simulink model "New_Control_Law_I_3Axis"  (R2016a)
settings: configuration reference "AR_Drone_ConfigSet" (kept outside this file)
values from neighbouring files (symbols this model uses):
  Accel_Calib_Gain = Simulink.Parameter    [AR_DRONE_SCRIPT.m]
  Accel_Calib_Offset = Simulink.Parameter    [AR_DRONE_SCRIPT.m]
undefined symbols (not defined in the file or in its folder): Drone_StateModeType, Mag_Calib_Gain_Vector, Mag_Calib_Offset_Vector, Navigation, Navigation_KF_Lib, sigbuilder_block
libraries: simulink x16, vrlib x7, aerolibtransform2 x5, AR_Drone_Sensors x2, AR_Drone_Actuators x2, aerolibutil x2, dspnetwork x2
(part 2 of 3)

== system New_Control_Law_I_3Axis/Flight Controller/Supervisory Flight Controller/Attitude_Control/Yaw Counter-Active Control ==
  note: This Yaw Controller will prevent the drone from
      | rotating but does not tell the drone to rotate to a specified angle
  Euler_Yaw_Deg : Inport
  Rate_Gyro_R_deg : Inport  Port=2
  "Desired_yaw " : Inport  Port=3
  Add1 : Sum  Inputs=+-  AccumDataTypeStr=single  OutDataTypeStr=single
  Add2 : Sum  Inputs=+-  AccumDataTypeStr=single  OutDataTypeStr=single
  Data Type Conversion : DataTypeConversion  OutDataTypeStr=int16
  Discrete Derivative : simulink/Discrete/Discrete Derivative  gainval=1.0  ICPrevScaledInput=0.0  InputProcessing=Inherited  OutMin=[]  OutMax=[]  OutDataType=fixdt(1, 16)  OutScaling=2^-10  DoSatur=off
  InterChange_Axis : Gain  Gain=-1  ParamDataTypeStr=single  OutDataTypeStr=single
      settings: AttributesFormatString=%<Gain>
  To Degrees2 : Gain  Gain=180/pi  ParamDataTypeStr=single  OutDataTypeStr=single
      settings: AttributesFormatString=%<Gain>
  To Degrees3 : Gain  ParamDataTypeStr=single  OutDataTypeStr=single
      settings: AttributesFormatString=%<Gain>
  Yaw_contribution : Gain  Gain=2.5*2  ParamDataTypeStr=single  OutDataTypeStr=single
      settings: AttributesFormatString=%<Gain>
  Yaw_contribution1 : Gain  Gain=0.04  ParamDataTypeStr=single  OutDataTypeStr=single
      settings: AttributesFormatString=%<Gain>
  YawCommand : Outport
  wires:
  Yaw_contribution1/1 -> Data Type Conversion/1
  To Degrees3/1 -> Add1/2
  Euler_Yaw_Deg/1 -> InterChange_Axis/1
  Add1/1 -> Yaw_contribution1/1
  Yaw_contribution/1 -> Add1/1
  Add2/1 -> Yaw_contribution/1
  InterChange_Axis/1 -> Discrete Derivative/1
  Discrete Derivative/1 -> Add2/1
  To Degrees2/1 -> Add2/2
  "Desired_yaw "/1 -> To Degrees2/1
  Rate_Gyro_R_deg/1 -> To Degrees3/1
  Data Type Conversion/1 -> YawCommand/1

== system New_Control_Law_I_3Axis/Flight Controller/Supervisory Flight Controller/Attitude_Control/Yaw Signal Builder  ==
  Demux : Demux  Tag=STV Demux  Outputs=1
  FromWs : FromWorkspace  Tag=STV FromWs  VariableName=tuvar
      SigBuilderData=|
      | common.afterFinalStr = 'Extrapolate'
      | common.sampleTime = '-1'
      | dataSet.timeRange = [0 20]
      | dataSet.name = 'Group 1'
      | sbobj.Groups.Name = 'Group 1'
      | sbobj.Groups.Signals.Name = 'Signal 1'
      | sbobj.Groups.Signals.XData = [0 10 10 12.5 12.5 15 15 20]
      | sbobj.Groups.Signals.YData = [0 0 2 2 -2 -2 0 0]
      | sbobj.Groups.TimeRange = [0 20]
  Signal 1 : Outport  Tag=STV Outport
  wires:
  Demux/1 -> Signal 1/1
  FromWs/1 -> Demux/1

== system New_Control_Law_I_3Axis/Navigation/CheckSum Pre-Processing/Accelerometer Processing ==
  Raw Data : Inport
  CheckSum Flag : Inport  Port=2
  Holding Value : Inport  Port=3
  Calculate Accel Data : Subsystem  Commented=through
  CheckSum Correction : Subsystem
  Processed Data : Outport
  wires:
  Holding Value/1 -> CheckSum Correction/3(Holding Value)
  Calculate Accel Data/1(Processed Accel Data) -> CheckSum Correction/1(CalculatedData)
  CheckSum Correction/1(Pre-Processed Height) -> Processed Data/1
  Raw Data/1 -> Calculate Accel Data/1(Raw Accel Data)
  CheckSum Flag/1 -> CheckSum Correction/2(CheckSumFlag)

== system New_Control_Law_I_3Axis/Navigation/CheckSum Pre-Processing/Magnetometer ==
  Magnetometer : Inport
  CheckSum Flag : Inport  Port=2
  Holding Value : Inport  Port=3
  CheckSum Correction : Subsystem
  Process Raw Mag Data : Subsystem  Commented=through
  Processed Data : Outport
  wires:
  Holding Value/1 -> CheckSum Correction/3(Holding Value)
  Process Raw Mag Data/1(ProcessedData) -> CheckSum Correction/1(CalculatedData)
  Magnetometer/1 -> Process Raw Mag Data/1(Magnetometer)
  CheckSum Correction/1(Pre-Processed Data) -> Processed Data/1
  CheckSum Flag/1 -> CheckSum Correction/2(CheckSumFlag)

== system New_Control_Law_I_3Axis/Navigation/CheckSum Pre-Processing/RateGyro Processing ==
  Raw Data : Inport
  CheckSum Flag : Inport  Port=2
  Holding Value : Inport  Port=3
  CheckSum Correction : Subsystem
  Process Data : Subsystem  Commented=through
  Processed Data : Outport
  wires:
  Holding Value/1 -> CheckSum Correction/3(Holding Value)
  Process Data/1(Processed Data) -> CheckSum Correction/1(CalculatedData)
  Raw Data/1 -> Process Data/1(Raw Data)
  CheckSum Correction/1(Pre-Processed Height) -> Processed Data/1
  CheckSum Flag/1 -> CheckSum Correction/2(CheckSumFlag)

== system New_Control_Law_I_3Axis/Navigation/CheckSum Pre-Processing/TempFilter ==
  Magnetometer : Inport
  CheckSum Flag : Inport  Port=2
  HoldingValue : Inport  Port=3
  CheckSum Correction : Subsystem
  Process Raw Mag Data : Subsystem  Commented=through
  Processed Data : Outport
  wires:
  HoldingValue/1 -> CheckSum Correction/3(Holding Value)
  Process Raw Mag Data/1(ProcessedData) -> CheckSum Correction/1(CalculatedData)
  Magnetometer/1 -> Process Raw Mag Data/1(Magnetometer)
  CheckSum Correction/1(Pre-Processed Data) -> Processed Data/1
  CheckSum Flag/1 -> CheckSum Correction/2(CheckSumFlag)

== system New_Control_Law_I_3Axis/Navigation/CheckSum Pre-Processing/Ultrasound Processing ==
  note: '192.168.1.1' 1 17725
  Raw Ultrasound : Inport
  CheckSum Flag : Inport  Port=2
  Holding Value : Inport  Port=3
  CheckSum Correction : Subsystem
  Data Type Conversion1 : DataTypeConversion
  Delay1 : Delay  DelayLength=1  InitialCondition=0
  Height Calculation : MATLAB Function  TreatAsAtomicUnit=on
  Saturation1 : Saturate  UpperLimit=100e3  LowerLimit=0
  Processed Data : Outport
  wires:
  Holding Value/1 -> CheckSum Correction/3(Holding Value)
  Saturation1/1 -> Processed Data/1
  CheckSum Correction/1(Pre-Processed Height) -> Saturation1/1
  CheckSum Flag/1 -> CheckSum Correction/2(CheckSumFlag)
  Height Calculation/1(y) -> CheckSum Correction/1(CalculatedData)
  Raw Ultrasound/1 -> Data Type Conversion1/1
  Height Calculation/2(prev_good_height) -> Delay1/1
  Data Type Conversion1/1 -> Height Calculation/1(u)
  Delay1/1 -> Height Calculation/2(z_1)

== system New_Control_Law_I_3Axis/Navigation/Data Conversion and Measurement Calculation/Calculate Gravity Vector ==
  Accel : Inport
  Accel_Offset : Inport  Port=2
  Accelerometer Neutral Gain and Offset : Subsystem
  Calibration_GainOffset : Subsystem
  Compare Calibration : Scope  NumInputPorts=2
  Compare Filter : Scope  NumInputPorts=2
  Compare Offset : Scope  NumInputPorts=2
  InitialCondition_Offset : Subsystem
  Low Pass Filter : Subsystem
  Normalize Vector : vrlib/Utilities/Normalize Vector  maxzero=0
  Accel_Norm : Outport
  wires:
  Accel_Offset/1 -> InitialCondition_Offset/2(Accel_Offset)
  Accelerometer Neutral Gain and Offset/1(Processed Accel Data) -> Compare Calibration/2, Calibration_GainOffset/1(Pre)
  Calibration_GainOffset/1(Post) -> Compare Offset/2, Compare Calibration/1, InitialCondition_Offset/1(Pre)
  Low Pass Filter/1(Filtered Accel) -> Normalize Vector/1, Compare Filter/1
  InitialCondition_Offset/1(Post) -> Low Pass Filter/1(Offset Accel), Compare Filter/2, Compare Offset/1
  Accel/1 -> Accelerometer Neutral Gain and Offset/1(Raw Accel Data)
  Normalize Vector/1 -> Accel_Norm/1

== system New_Control_Law_I_3Axis/Navigation/Data Conversion and Measurement Calculation/Calibration_Scale_and_Offset ==
  RawMag : Inport
  Normalize Vector : vrlib/Utilities/Normalize Vector  maxzero=0
  Process Raw Mag Data : Subsystem  Variant=on  OverrideUsingVariant=TempVariantA
  Normalized  Magnetometer : Outport
  wires:
  Process Raw Mag Data/1(MagVector) -> Normalize Vector/1
  RawMag/1 -> Process Raw Mag Data/1(Magnetometer)
  Normalize Vector/1 -> Normalized  Magnetometer/1

== system New_Control_Law_I_3Axis/Navigation/Data Conversion and Measurement Calculation/Remove Offset ==
  Raw Gyro Values : Inport
  Gyro Offset : Inport  Port=2
  BeforeAfter : Scope
  Demux : Demux  Outputs=3
  Demux1 : Demux  Outputs=3
  Display : Display
  Mux : Mux  Inputs=2
  Mux1 : Mux  Inputs=3
  Process Raw Rate Gyro Data : Subsystem
  Sum : Sum  Inputs=|+-
  Sum1 : Sum  Inputs=|+-
  Sum2 : Sum  Inputs=|+-
  Gyro Offset Remove : Outport
  tag scope: GyroOffset_Tag=global
  wires:
  Process Raw Rate Gyro Data/1(Processed Data) -> Gyro Offset Remove/1
  Mux/1 -> BeforeAfter/1
  Raw Gyro Values/1 -> Demux/1, Mux/1, [GyroOffset_Tag]
  Gyro Offset/1 -> Demux1/1
  Mux1/1 -> Process Raw Rate Gyro Data/1(Raw Rate Gyro Data), Display/1, Mux/2
  Demux1/3 -> Sum2/2
  Demux1/2 -> Sum1/2
  Demux1/1 -> Sum/2
  Demux/2 -> Sum1/1
  Demux/1 -> Sum/1
  Sum1/1 -> Mux1/2
  Demux/3 -> Sum2/1
  Sum2/1 -> Mux1/3
  Sum/1 -> Mux1/1

== system New_Control_Law_I_3Axis/Navigation/SL3D Visualization/Interchange Axes Accel for SL3D  ==
  VRML_in : Inport
  Demux1 : Demux  Outputs=3
  Gain1 : Gain  Gain=3
  Gain2 : Gain
  Gain3 : Gain
  Mux2 : Mux  Inputs=3
  VRML_out : Outport
  wires:
  VRML_in/1 -> Gain1/1
  Demux1/2 -> Gain2/1
  Mux2/1 -> VRML_out/1
  Gain3/1 -> Mux2/3
  Gain2/1 -> Mux2/1
  Demux1/3 -> Mux2/2
  Demux1/1 -> Gain3/1
  Gain1/1 -> Demux1/1

== system New_Control_Law_I_3Axis/Navigation/SL3D Visualization/Interchange Axes Mag for SL3D  ==
  VRML_in : Inport
  Home Drone : Subsystem
  Subsystem : Subsystem  Commented=on
  Work Drone : Subsystem
  Work Drone - supposed work drone .. not really : Subsystem
  VRML_out : Outport
  wires:
  Work Drone/1(Out1) -> VRML_out/1
  VRML_in/1 -> Home Drone/1(In1), Work Drone/1(In1)

== system New_Control_Law_I_3Axis/Navigation/SL3D Visualization/Interchange Axis Mag Project for SL3D ==
  VRML_in : Inport
  Demux1 : Demux  Outputs=3
  Gain2 : Gain
  Gain3 : Gain
  Mux2 : Mux  Inputs=3
  VRML_out : Outport
  wires:
  Demux1/2 -> Gain2/1
  Mux2/1 -> VRML_out/1
  Gain3/1 -> Mux2/3
  Gain2/1 -> Mux2/1
  Demux1/3 -> Mux2/2
  Demux1/1 -> Gain3/1
  VRML_in/1 -> Demux1/1

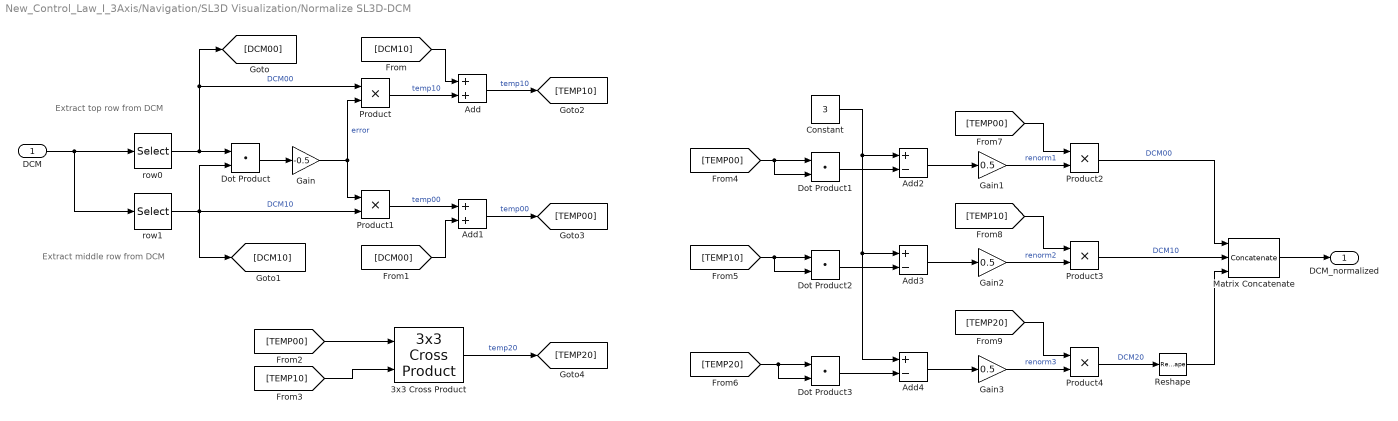
== system New_Control_Law_I_3Axis/Navigation/SL3D Visualization/Normalize SL3D-DCM ==
  note: Extract top row from DCM
  note: Extract middle row from DCM
  DCM : Inport  OutDataTypeStr=double  PortDimensions=[3,3]
  3x3 Cross Product : aerolibutil/3x3 Cross Product
  Add : Sum
  Add1 : Sum
  Add2 : Sum  Inputs=+-
  Add3 : Sum  Inputs=+-
  Add4 : Sum  Inputs=+-
  Constant : Constant  Value=3  OutDataTypeStr=double  SampleTime=-1
  Dot Product{,1..3} (4 alike) : DotProduct  InputSameDT=on  OutDataTypeStr=Inherit: Inherit via internal rule
  Gain : Gain  Gain=-0.5
  Gain1 : Gain  Gain=0.5  OutDataTypeStr=single
  Gain2 : Gain  Gain=0.5  OutDataTypeStr=single
  Gain3 : Gain  Gain=0.5  OutDataTypeStr=single
  Matrix Concatenate : Concatenate  NumInputs=3  Mode=Multidimensional array
  Product{,1..4} (5 alike) : Product  RndMeth=Zero
  Reshape : Reshape  OutputDimensionality=Row vector (2-D)
  row0 : Selector  NumberOfDimensions=2  IndexMode=Zero-based  InputPortWidth=3  IndexOptions=Index vector (dialog),Index vector (dialog)  Indices=0,[0:2]  OutputSizes=1,1
  row1 : Selector  NumberOfDimensions=2  IndexMode=Zero-based  InputPortWidth=3  IndexOptions=Index vector (dialog),Index vector (dialog)  Indices=1,[0:2]  OutputSizes=1,1
  DCM_normalized : Outport  OutDataTypeStr=double
  wires:
  DCM/1 -> row0/1, row1/1
  row0/1 -> Dot Product/1, Product/1, [DCM00]  "DCM00"
  row1/1 -> Dot Product/2, Product1/2, [DCM10]  "DCM10"
  Dot Product/1 -> Gain/1
  Gain/1 -> Product/2, Product1/1  "error"
  Product/1 -> Add/2  "temp10"
  Product1/1 -> Add1/1  "temp00"
  [DCM10] -> Add/1
  [DCM00] -> Add1/2
  Add/1 -> [TEMP10]  "temp10"
  Add1/1 -> [TEMP00]  "temp00"
  3x3 Cross Product/1 -> [TEMP20]  "temp20"
  [TEMP00] -> 3x3 Cross Product/1
  [TEMP10] -> 3x3 Cross Product/2
  [TEMP00] -> Dot Product1/1, Dot Product1/2
  [TEMP10] -> Dot Product2/1, Dot Product2/2
  [TEMP20] -> Dot Product3/1, Dot Product3/2
  Dot Product1/1 -> Add2/2
  Constant/1 -> Add2/1, Add4/1, Add3/1
  Add2/1 -> Gain1/1
  Gain1/1 -> Product2/2  "renorm1"
  Add3/1 -> Gain2/1
  Gain2/1 -> Product3/2  "renorm2"
  Dot Product2/1 -> Add3/2
  Add4/1 -> Gain3/1
  Gain3/1 -> Product4/2  "renorm3"
  Dot Product3/1 -> Add4/2
  [TEMP00] -> Product2/1
  [TEMP10] -> Product3/1
  [TEMP20] -> Product4/1
  Product2/1 -> Matrix Concatenate/1  "DCM00"
  Product3/1 -> Matrix Concatenate/2  "DCM10"
  Product4/1 -> Reshape/1  "DCM20"
  Matrix Concatenate/1 -> DCM_normalized/1
  Reshape/1 -> Matrix Concatenate/3

== system New_Control_Law_I_3Axis/Navigation/SL3D Visualization/SL3D DCM Output - used to adjust axes to fit wit SL3D convention ==

== system New_Control_Law_I_3Axis/SL3D Visualization/Interchange Axes Mag for SL3D /Home Drone ==
  note: z
  note: x
  note: y
  note: This comes close, however, it doesnt seem that the axis changes properly
      | ie: i rotate drone, the green dot follows it. This  tells me the Z-axis is not
      |  properly placed
  In1 : Inport
  Demux1 : Demux  Outputs=3
  Gain : Gain  Gain=-1
  Gain1 : Gain
  Gain2 : Gain
  Mux2 : Mux  Inputs=3
  Out1 : Outport
  wires:
  Gain1/1 -> Mux2/1
  Demux1/2 -> Gain1/1
  Gain/1 -> Mux2/3
  Demux1/1 -> Gain/1
  Gain2/1 -> Mux2/2
  Demux1/3 -> Gain2/1
  In1/1 -> Demux1/1
  Mux2/1 -> Out1/1

== system New_Control_Law_I_3Axis/SL3D Visualization/Interchange Axes Mag for SL3D /Subsystem ==
  note: z
  note: x
  note: y
  note: This comes close, however, it doesnt seem that the axis changes properly
      | ie: i rotate drone, the green dot follows it. This  tells me the Z-axis is not
      |  properly placed
  In1 : Inport
  Demux1 : Demux  Outputs=3
  Gain : Gain
  Gain1 : Gain  Gain=-1
  Gain2 : Gain  Gain=-1
  Mux2 : Mux  Inputs=3
  Out1 : Outport
  wires:
  In1/1 -> Demux1/1
  Demux1/3 -> Gain/1
  Demux1/2 -> Gain1/1
  Mux2/1 -> Out1/1
  Gain1/1 -> Mux2/1
  Gain/1 -> Mux2/3
  Gain2/1 -> Mux2/2
  Demux1/1 -> Gain2/1

== system New_Control_Law_I_3Axis/SL3D Visualization/Interchange Axes Mag for SL3D /Work Drone ==
  note: z
  note: x
  note: y
  note: This comes close, however, it doesnt seem that the axis changes properly
      | ie: i rotate drone, the green dot follows it. This  tells me the Z-axis is not
      |  properly placed
  In1 : Inport
  Demux1 : Demux  Outputs=3
  Gain : Gain  Gain=-1
  Gain1 : Gain
  Gain2 : Gain
  Mux2 : Mux  Inputs=3
  Out1 : Outport
  wires:
  Gain1/1 -> Mux2/1
  Demux1/2 -> Gain1/1
  Gain/1 -> Mux2/3
  Demux1/1 -> Gain/1
  Gain2/1 -> Mux2/2
  Demux1/3 -> Gain2/1
  In1/1 -> Demux1/1
  Mux2/1 -> Out1/1

== system New_Control_Law_I_3Axis/SL3D Visualization/Interchange Axes Mag for SL3D /Work Drone - supposed work drone .. not really ==
  note: z
  note: x
  note: y
  note: This comes close, however, it doesnt seem that the axis changes properly
      | ie: i rotate drone, the green dot follows it. This  tells me the Z-axis is not
      |  properly placed
  In1 : Inport
  Demux1 : Demux  Outputs=3
  Gain : Gain  Gain=-1
  Gain1 : Gain
  Gain2 : Gain  Gain=-1
  Mux2 : Mux  Inputs=3
  Out1 : Outport
  wires:
  Gain1/1 -> Mux2/1
  Demux1/2 -> Gain1/1
  Gain/1 -> Mux2/3
  Demux1/1 -> Gain/1
  Gain2/1 -> Mux2/2
  Demux1/3 -> Gain2/1
  In1/1 -> Demux1/1
  Mux2/1 -> Out1/1

== system New_Control_Law_I_3Axis/Sensor  Telemetry/CheckSum_Correct_Pressure/CheckSum Correction ==
  CalculatedData : Inport
  CheckSumFlag : Inport  Port=2
  Holding Value : Inport  Port=3
  Compare To Zero : simulink/Logic and Bit Operations/Compare To Zero  relop=>  OutDataTypeStr=boolean
  Delay : Delay  DelayLength=3  InitialCondition=0
  Generate Sample Holding Pulse : Subsystem
  "If True, we have good data, If false, we have bad data, With bad data, use previous good data from N samples ago and hold it on that value for M samples" : Switch  Criteria=u2 > Threshold
  Invert Logic : Logic  Operator=NOT  AllPortsSameDT=off  OutDataTypeStr=boolean
  Logical Operator1 : Logic  Operator=NOT  AllPortsSameDT=off  OutDataTypeStr=boolean
  Pre-Processed Height : Outport
  wires:
  CheckSumFlag/1 -> Compare To Zero/1
  CalculatedData/1 -> "If True, we have good data, If false, we have bad data, With bad data, use previous good data from N samples ago and hold it on that value for M samples"/1
  "If True, we have good data, If false, we have bad data, With bad data, use previous good data from N samples ago and hold it on that value for M samples"/1 -> Pre-Processed Height/1, Delay/1
  Delay/1 -> "If True, we have good data, If false, we have bad data, With bad data, use previous good data from N samples ago and hold it on that value for M samples"/3
  Compare To Zero/1 -> Logical Operator1/1
  Generate Sample Holding Pulse/1(Hold_Data_Pulse) -> Invert Logic/1
  Logical Operator1/1 -> Generate Sample Holding Pulse/1(CheckSumFlag)
  Invert Logic/1 -> "If True, we have good data, If false, we have bad data, With bad data, use previous good data from N samples ago and hold it on that value for M samples"/2
  Holding Value/1 -> Generate Sample Holding Pulse/2(HoldDataTicks_Value)

== system New_Control_Law_I_3Axis/Sensor  Telemetry/CheckSum_Correct_Temp/CheckSum Correction ==
  CalculatedData : Inport
  CheckSumFlag : Inport  Port=2
  Holding Value : Inport  Port=3
  Compare To Zero : simulink/Logic and Bit Operations/Compare To Zero  relop=>  OutDataTypeStr=boolean
  Delay : Delay  DelayLength=3  InitialCondition=0
  Generate Sample Holding Pulse : Subsystem
  "If True, we have good data, If false, we have bad data, With bad data, use previous good data from N samples ago and hold it on that value for M samples" : Switch  Criteria=u2 > Threshold
  Invert Logic : Logic  Operator=NOT  AllPortsSameDT=off  OutDataTypeStr=boolean
  Logical Operator1 : Logic  Operator=NOT  AllPortsSameDT=off  OutDataTypeStr=boolean
  Pre-Processed Height : Outport
  wires:
  CheckSumFlag/1 -> Compare To Zero/1
  CalculatedData/1 -> "If True, we have good data, If false, we have bad data, With bad data, use previous good data from N samples ago and hold it on that value for M samples"/1
  "If True, we have good data, If false, we have bad data, With bad data, use previous good data from N samples ago and hold it on that value for M samples"/1 -> Pre-Processed Height/1, Delay/1
  Delay/1 -> "If True, we have good data, If false, we have bad data, With bad data, use previous good data from N samples ago and hold it on that value for M samples"/3
  Compare To Zero/1 -> Logical Operator1/1
  Generate Sample Holding Pulse/1(Hold_Data_Pulse) -> Invert Logic/1
  Logical Operator1/1 -> Generate Sample Holding Pulse/1(CheckSumFlag)
  Invert Logic/1 -> "If True, we have good data, If false, we have bad data, With bad data, use previous good data from N samples ago and hold it on that value for M samples"/2
  Holding Value/1 -> Generate Sample Holding Pulse/2(HoldDataTicks_Value)

== system New_Control_Law_I_3Axis/Sensor  Telemetry/Data Collection/Low Pass Filter ==
  GyroMeasure : Inport
  Demux : Demux  Outputs=2
  Digital Low Pass Filter1 : DiscreteTransferFcn  Numerator=[0.04877]  Denominator=[1 -0.9512]  OutDataTypeStr=int16
  Digital Low Pass Filter2 : DiscreteTransferFcn  Numerator=[0.04877]  Denominator=[1 -0.9512]  OutDataTypeStr=int16
  Digital Low Pass Filter3 : DiscreteTransferFcn  Commented=on  Numerator=[0.04877]  Denominator=[1 -0.9512]  OutDataTypeStr=int16
  Mux3 : Mux  Inputs=2
  GyroFiltered : Outport
  wires:
  Mux3/1 -> GyroFiltered/1
  Demux/1 -> Digital Low Pass Filter2/1
  GyroMeasure/1 -> Demux/1
  Demux/2 -> Digital Low Pass Filter1/1
  Digital Low Pass Filter2/1 -> Mux3/1
  Digital Low Pass Filter1/1 -> Mux3/2

== system New_Control_Law_I_3Axis/Flight Controller/Supervisory Flight Controller/Attitude_Control/Roll Pitch Controller/Low Pass Filter ==
  GyroMeasure : Inport
  Demux : Demux  Outputs=2
  Digital Low Pass Filter1 : DiscreteTransferFcn  Numerator=[0.04877]  Denominator=[1 -0.9512]  OutDataTypeStr=int16
  Digital Low Pass Filter2 : DiscreteTransferFcn  Numerator=[0.04877]  Denominator=[1 -0.9512]  OutDataTypeStr=int16
  Digital Low Pass Filter3 : DiscreteTransferFcn  Commented=on  Numerator=[0.04877]  Denominator=[1 -0.9512]  OutDataTypeStr=int16
  Mux3 : Mux  Inputs=2
  GyroFiltered : Outport
  wires:
  Mux3/1 -> GyroFiltered/1
  Demux/1 -> Digital Low Pass Filter2/1
  GyroMeasure/1 -> Demux/1
  Demux/2 -> Digital Low Pass Filter1/1
  Digital Low Pass Filter2/1 -> Mux3/1
  Digital Low Pass Filter1/1 -> Mux3/2

== system New_Control_Law_I_3Axis/Flight Controller/Supervisory Flight Controller/Attitude_Control/Roll Pitch Controller/Outer Loop Euler Angle Control Loop ==
  Attitude_Rate : Inport
  Motor Armed : Inport  Port=2
  Logical Operator : Logic  Operator=NOT  AllPortsSameDT=off  OutDataTypeStr=boolean
  PID Controller : simulink/Continuous/PID Controller  Controller=PID  TimeDomain=Discrete-time  SampleTime=-1  IntegratorMethod=Forward Euler  FilterMethod=Forward Euler  Form=Parallel  UseFilter=on  ControllerParametersSource=internal  P=2.8281  I=28.23  D=0.023379  N=0.0076593  InitialConditionSource=internal  InitialConditionForIntegrator=0  InitialConditionForFilter=0  ExternalReset=level  LimitOutput=on  UpperSaturationLimit=30  LowerSaturationLimit=-30  LinearizeAsGain=on  AntiWindupMode=clamping  Kb=1  TrackingMode=off  Kt=1  PParamMin=[]  PParamMax=[]  IParamMin=[]  IParamMax=[]  DParamMin=[]  DParamMax=[]  NParamMin=[]  NParamMax=[]  KbParamMin=[]  KbParamMax=[]  KtParamMin=[]  KtParamMax=[]  POutMin=[]  POutMax=[]  IOutMin=[]  IOutMax=[]  DOutMin=[]  DOutMax=[]  NOutMin=[]  NOutMax=[]  KbOutMin=[]  KbOutMax=[]  KtOutMin=[]  KtOutMax=[]  IntegratorOutMin=[]  IntegratorOutMax=[]  FilterOutMin=[]  FilterOutMax=[]  SumOutMin=[]  SumOutMax=[]  SumI1OutMin=[]  SumI1OutMax=[]  SumI2OutMin=[]  SumI2OutMax=[]  SumI3OutMin=[]  SumI3OutMax=[]  SumDOutMin=[]  SumDOutMax=[]  SaturationOutMin=[]  SaturationOutMax=[]  IntegratorContinuousStateAttributes=''  IntegratorStateMustResolveToSignalObject=off  IntegratorRTWStateStorageClass=Auto  FilterContinuousStateAttributes=''  FilterStateMustResolveToSignalObject=off  FilterRTWStateStorageClass=Auto  DifferentiatorICPrevScaledInput=0  DifferentiatorOutMin=[]  DifferentiatorOutMax=[]
  PID Controller1 : simulink/Continuous/PID Controller  Controller=PID  TimeDomain=Discrete-time  SampleTime=-1  IntegratorMethod=Forward Euler  FilterMethod=Forward Euler  Form=Parallel  UseFilter=on  ControllerParametersSource=internal  P=0.10084*2  I=0.13631*2  D=-0.011755  N=5  InitialConditionSource=internal  InitialConditionForIntegrator=0  InitialConditionForFilter=0  ExternalReset=level  LimitOutput=on  UpperSaturationLimit=30  LowerSaturationLimit=-30  LinearizeAsGain=on  AntiWindupMode=clamping  Kb=1  TrackingMode=off  Kt=1  PParamMin=[]  PParamMax=[]  IParamMin=[]  IParamMax=[]  DParamMin=[]  DParamMax=[]  NParamMin=[]  NParamMax=[]  KbParamMin=[]  KbParamMax=[]  KtParamMin=[]  KtParamMax=[]  POutMin=[]  POutMax=[]  IOutMin=[]  IOutMax=[]  DOutMin=[]  DOutMax=[]  NOutMin=[]  NOutMax=[]  KbOutMin=[]  KbOutMax=[]  KtOutMin=[]  KtOutMax=[]  IntegratorOutMin=[]  IntegratorOutMax=[]  FilterOutMin=[]  FilterOutMax=[]  SumOutMin=[]  SumOutMax=[]  SumI1OutMin=[]  SumI1OutMax=[]  SumI2OutMin=[]  SumI2OutMax=[]  SumI3OutMin=[]  SumI3OutMax=[]  SumDOutMin=[]  SumDOutMax=[]  SaturationOutMin=[]  SaturationOutMax=[]  IntegratorContinuousStateAttributes=''  IntegratorStateMustResolveToSignalObject=off  IntegratorRTWStateStorageClass=Auto  FilterContinuousStateAttributes=''  FilterStateMustResolveToSignalObject=off  FilterRTWStateStorageClass=Auto  DifferentiatorICPrevScaledInput=0  DifferentiatorOutMin=[]  DifferentiatorOutMax=[]
  AttitudeRateCmd : Outport
  wires:
  PID Controller1/1 -> AttitudeRateCmd/1  "AttitudeRateCmd"
  Motor Armed/1 -> Logical Operator/1
  Logical Operator/1 -> PID Controller1/2
  Attitude_Rate/1 -> PID Controller1/1

== system New_Control_Law_I_3Axis/Navigation/CheckSum Pre-Processing/Accelerometer Processing/Calculate Accel Data ==
  Raw Accel Data : Inport
  Bias : Constant  Value=[0 4096 4096]
  Gain : Gain  Gain=[0.001953125, 0.001953125, 0.001953125]
  Neutral Bias : Constant  Value=[2048 2048 2048]
  Sum : Sum  Inputs=|-+
  Sum1 : Sum  Inputs=|+-
  Processed Accel Data : Outport
  wires:
  Bias/1 -> Sum/2
  Neutral Bias/1 -> Sum1/2
  Sum/1 -> Sum1/1
  Gain/1 -> Processed Accel Data/1
  Sum1/1 -> Gain/1
  Raw Accel Data/1 -> Sum/1

== system New_Control_Law_I_3Axis/Navigation/CheckSum Pre-Processing/Accelerometer Processing/CheckSum Correction ==
  CalculatedData : Inport
  CheckSumFlag : Inport  Port=2
  Holding Value : Inport  Port=3
  Compare To Zero : simulink/Logic and Bit Operations/Compare To Zero  relop=>  OutDataTypeStr=boolean
  Delay : Delay  DelayLength=3  InitialCondition=0
  Generate Sample Holding Pulse : Subsystem
  "If True, we have good data, If false, we have bad data, With bad data, use previous good data from N samples ago and hold it on that value for M samples" : Switch  Criteria=u2 > Threshold
  Invert Logic : Logic  Operator=NOT  AllPortsSameDT=off  OutDataTypeStr=boolean
  Logical Operator1 : Logic  Operator=NOT  AllPortsSameDT=off  OutDataTypeStr=boolean
  Pre-Processed Height : Outport
  wires:
  Holding Value/1 -> Generate Sample Holding Pulse/2(HoldDataTicks_Value)
  Invert Logic/1 -> "If True, we have good data, If false, we have bad data, With bad data, use previous good data from N samples ago and hold it on that value for M samples"/2
  Logical Operator1/1 -> Generate Sample Holding Pulse/1(CheckSumFlag)
  Generate Sample Holding Pulse/1(Hold_Data_Pulse) -> Invert Logic/1
  Compare To Zero/1 -> Logical Operator1/1
  Delay/1 -> "If True, we have good data, If false, we have bad data, With bad data, use previous good data from N samples ago and hold it on that value for M samples"/3
  "If True, we have good data, If false, we have bad data, With bad data, use previous good data from N samples ago and hold it on that value for M samples"/1 -> Delay/1, Pre-Processed Height/1
  CalculatedData/1 -> "If True, we have good data, If false, we have bad data, With bad data, use previous good data from N samples ago and hold it on that value for M samples"/1
  CheckSumFlag/1 -> Compare To Zero/1

== system New_Control_Law_I_3Axis/Navigation/CheckSum Pre-Processing/Magnetometer/CheckSum Correction ==
  CalculatedData : Inport
  CheckSumFlag : Inport  Port=2
  Holding Value : Inport  Port=3
  Compare To Zero : simulink/Logic and Bit Operations/Compare To Zero  relop=>  OutDataTypeStr=boolean
  Delay : Delay  DelayLength=3  InitialCondition=0
  Generate Sample Holding Pulse : Subsystem
  "If True, we have good data, If false, we have bad data, With bad data, use previous good data from N samples ago and hold it on that value for M samples" : Switch  Criteria=u2 > Threshold
  Invert Logic : Logic  Operator=NOT  AllPortsSameDT=off  OutDataTypeStr=boolean
  Logical Operator1 : Logic  Operator=NOT  AllPortsSameDT=off  OutDataTypeStr=boolean
  Pre-Processed Data : Outport
  wires:
  Holding Value/1 -> Generate Sample Holding Pulse/2(HoldDataTicks_Value)
  Invert Logic/1 -> "If True, we have good data, If false, we have bad data, With bad data, use previous good data from N samples ago and hold it on that value for M samples"/2
  Logical Operator1/1 -> Generate Sample Holding Pulse/1(CheckSumFlag)
  Generate Sample Holding Pulse/1(Hold_Data_Pulse) -> Invert Logic/1
  Compare To Zero/1 -> Logical Operator1/1
  Delay/1 -> "If True, we have good data, If false, we have bad data, With bad data, use previous good data from N samples ago and hold it on that value for M samples"/3
  "If True, we have good data, If false, we have bad data, With bad data, use previous good data from N samples ago and hold it on that value for M samples"/1 -> Delay/1, Pre-Processed Data/1
  CalculatedData/1 -> "If True, we have good data, If false, we have bad data, With bad data, use previous good data from N samples ago and hold it on that value for M samples"/1
  CheckSumFlag/1 -> Compare To Zero/1

== system New_Control_Law_I_3Axis/Navigation/CheckSum Pre-Processing/Magnetometer/Process Raw Mag Data ==
  note: magnetometer[ 0 ] = - ( float ) navdata.mx ;
      | magnetometer[ 1 ] = ( float ) navdata.my ;
      | magnetometer[ 2 ] = - ( float ) navdata.mz ;
      | const float Sensitivity[ 3 ] = { 0.0071492608 , 0.0070882491 , 0.0074057781 } ;
      | const float Neutral[ 3 ] = { 118.0 , - 65.0 , 110.0 } ;
  Magnetometer : Inport
  Bias : Constant  Value=[ 118.0, -65.0, 110.0 ]
  Sum : Sum  Inputs=|+-
  postGain : Gain  Gain=[0.0071492608, 0.0070882491, 0.0074057781]
  preGain : Gain  Gain=[-1 1 -1]
  ProcessedData : Outport
  wires:
  Bias/1 -> Sum/2
  preGain/1 -> Sum/1
  Sum/1 -> postGain/1
  Magnetometer/1 -> preGain/1
  postGain/1 -> ProcessedData/1

== system New_Control_Law_I_3Axis/Navigation/CheckSum Pre-Processing/RateGyro Processing/CheckSum Correction ==
  CalculatedData : Inport
  CheckSumFlag : Inport  Port=2
  Holding Value : Inport  Port=3
  Compare To Zero : simulink/Logic and Bit Operations/Compare To Zero  relop=>  OutDataTypeStr=boolean
  Delay : Delay  DelayLength=3  InitialCondition=0
  Generate Sample Holding Pulse : Subsystem
  "If True, we have good data, If false, we have bad data, With bad data, use previous good data from N samples ago and hold it on that value for M samples" : Switch  Criteria=u2 > Threshold
  Invert Logic : Logic  Operator=NOT  AllPortsSameDT=off  OutDataTypeStr=boolean
  Logical Operator1 : Logic  Operator=NOT  AllPortsSameDT=off  OutDataTypeStr=boolean
  Pre-Processed Height : Outport
  wires:
  Holding Value/1 -> Generate Sample Holding Pulse/2(HoldDataTicks_Value)
  Invert Logic/1 -> "If True, we have good data, If false, we have bad data, With bad data, use previous good data from N samples ago and hold it on that value for M samples"/2
  Logical Operator1/1 -> Generate Sample Holding Pulse/1(CheckSumFlag)
  Generate Sample Holding Pulse/1(Hold_Data_Pulse) -> Invert Logic/1
  Compare To Zero/1 -> Logical Operator1/1
  Delay/1 -> "If True, we have good data, If false, we have bad data, With bad data, use previous good data from N samples ago and hold it on that value for M samples"/3
  "If True, we have good data, If false, we have bad data, With bad data, use previous good data from N samples ago and hold it on that value for M samples"/1 -> Delay/1, Pre-Processed Height/1
  CalculatedData/1 -> "If True, we have good data, If false, we have bad data, With bad data, use previous good data from N samples ago and hold it on that value for M samples"/1
  CheckSumFlag/1 -> Compare To Zero/1

== system New_Control_Law_I_3Axis/Navigation/CheckSum Pre-Processing/RateGyro Processing/Process Data ==
  note: const float Sensitivity[ 3 ] = { 0.0609 , 0.0609 , 0.0609 } ;
      | const float Neutral[ 3 ] = { 0.0 , 0.0 , 0.0 } ;
      | const int16_t Offset[ 3 ] = { - 73 , 14 , - 13 } ;
      | const int16_t Noises[ 3 ] = { 35 , 35 , 15 } ;
      |
      | int16_t vRaws[ 3 ] = {
      | Navdata :: IMU :: Gyroscope :: getRawX (),
      | Navdata :: IMU :: Gyroscope :: getRawY (),
      | Navdata :: IMU :: Gyroscope :: getRawZ ()
      | } ;
      |
      | gyroscope[i] = vRaws[i] * Gyroscope :: Sensitivity[i] * M_PI / 180.0 ;
  Raw Data : Inport
  Constant : Constant  Value=[0.0, 0.0, 0.0]
  Gain : Gain  Gain=[0.0609, 0.0609, 0.0609]
  Sum : Sum  Inputs=|++
  Processed Data : Outport
  wires:
  Raw Data/1 -> Sum/1
  Constant/1 -> Sum/2
  Gain/1 -> Processed Data/1
  Sum/1 -> Gain/1

== system New_Control_Law_I_3Axis/Navigation/CheckSum Pre-Processing/TempFilter/CheckSum Correction ==
  CalculatedData : Inport
  CheckSumFlag : Inport  Port=2
  Holding Value : Inport  Port=3
  Compare To Zero : simulink/Logic and Bit Operations/Compare To Zero  relop=>  OutDataTypeStr=boolean
  Delay : Delay  DelayLength=3  InitialCondition=0
  Generate Sample Holding Pulse : Subsystem
  "If True, we have good data, If false, we have bad data, With bad data, use previous good data from N samples ago and hold it on that value for M samples" : Switch  Criteria=u2 > Threshold
  Invert Logic : Logic  Operator=NOT  AllPortsSameDT=off  OutDataTypeStr=boolean
  Logical Operator1 : Logic  Operator=NOT  AllPortsSameDT=off  OutDataTypeStr=boolean
  Pre-Processed Data : Outport
  wires:
  Holding Value/1 -> Generate Sample Holding Pulse/2(HoldDataTicks_Value)
  Invert Logic/1 -> "If True, we have good data, If false, we have bad data, With bad data, use previous good data from N samples ago and hold it on that value for M samples"/2
  Logical Operator1/1 -> Generate Sample Holding Pulse/1(CheckSumFlag)
  Generate Sample Holding Pulse/1(Hold_Data_Pulse) -> Invert Logic/1
  Compare To Zero/1 -> Logical Operator1/1
  Delay/1 -> "If True, we have good data, If false, we have bad data, With bad data, use previous good data from N samples ago and hold it on that value for M samples"/3
  "If True, we have good data, If false, we have bad data, With bad data, use previous good data from N samples ago and hold it on that value for M samples"/1 -> Delay/1, Pre-Processed Data/1
  CalculatedData/1 -> "If True, we have good data, If false, we have bad data, With bad data, use previous good data from N samples ago and hold it on that value for M samples"/1
  CheckSumFlag/1 -> Compare To Zero/1

== system New_Control_Law_I_3Axis/Navigation/CheckSum Pre-Processing/TempFilter/Process Raw Mag Data ==
  note: magnetometer[ 0 ] = - ( float ) navdata.mx ;
      | magnetometer[ 1 ] = ( float ) navdata.my ;
      | magnetometer[ 2 ] = - ( float ) navdata.mz ;
      | const float Sensitivity[ 3 ] = { 0.0071492608 , 0.0070882491 , 0.0074057781 } ;
      | const float Neutral[ 3 ] = { 118.0 , - 65.0 , 110.0 } ;
  Magnetometer : Inport
  Bias : Constant  Value=[ 118.0, -65.0, 110.0 ]
  Sum : Sum  Inputs=|+-
  postGain : Gain  Gain=[0.0071492608, 0.0070882491, 0.0074057781]
  preGain : Gain  Gain=[-1 1 -1]
  ProcessedData : Outport
  wires:
  Bias/1 -> Sum/2
  preGain/1 -> Sum/1
  Sum/1 -> postGain/1
  Magnetometer/1 -> preGain/1
  postGain/1 -> ProcessedData/1

== system New_Control_Law_I_3Axis/Navigation/CheckSum Pre-Processing/Ultrasound Processing/CheckSum Correction ==
  CalculatedData : Inport
  CheckSumFlag : Inport  Port=2
  Holding Value : Inport  Port=3
  Compare To Zero : simulink/Logic and Bit Operations/Compare To Zero  relop=>  OutDataTypeStr=boolean
  Delay : Delay  DelayLength=3  InitialCondition=0
  Generate Sample Holding Pulse : Subsystem
  "If True, we have good data, If false, we have bad data, With bad data, use previous good data from N samples ago and hold it on that value for M samples" : Switch  Criteria=u2 > Threshold
  Invert Logic : Logic  Operator=NOT  AllPortsSameDT=off  OutDataTypeStr=boolean
  Logical Operator1 : Logic  Operator=NOT  AllPortsSameDT=off  OutDataTypeStr=boolean
  Pre-Processed Height : Outport
  wires:
  Holding Value/1 -> Generate Sample Holding Pulse/2(HoldDataTicks_Value)
  Invert Logic/1 -> "If True, we have good data, If false, we have bad data, With bad data, use previous good data from N samples ago and hold it on that value for M samples"/2
  Logical Operator1/1 -> Generate Sample Holding Pulse/1(CheckSumFlag)
  Generate Sample Holding Pulse/1(Hold_Data_Pulse) -> Invert Logic/1
  Compare To Zero/1 -> Logical Operator1/1
  Delay/1 -> "If True, we have good data, If false, we have bad data, With bad data, use previous good data from N samples ago and hold it on that value for M samples"/3
  "If True, we have good data, If false, we have bad data, With bad data, use previous good data from N samples ago and hold it on that value for M samples"/1 -> Delay/1, Pre-Processed Height/1
  CalculatedData/1 -> "If True, we have good data, If false, we have bad data, With bad data, use previous good data from N samples ago and hold it on that value for M samples"/1
  CheckSumFlag/1 -> Compare To Zero/1

== system New_Control_Law_I_3Axis/Navigation/Data Conversion and Measurement Calculation/Calculate Gravity Vector/Accelerometer Neutral Gain and Offset ==
  note: (1/512)g /LSB
  note: All axes were invereted here, both implementations in paparazzi and student team seem to do this
  Raw Accel Data : Inport
  Bias : Constant  Value=[4096]
  Data Type Conversion : DataTypeConversion  OutDataTypeStr=int16
  Demux : Demux  Outputs=3
  Gain : Gain  Gain=1/512
  Gain1 : Gain  Gain=-1  OutDataTypeStr=double
  Gain2 : Gain  Gain=-1  OutDataTypeStr=double
  Gain3 : Gain  Gain=-1  OutDataTypeStr=double
  Mux : Mux  Inputs=3
  Neutral Bias : Constant  Value=[2048 2048 2048]
  Sum : Sum  Inputs=|++
  Sum1 : Sum  Inputs=|+-
  Sum2 : Sum  Inputs=|++
  Sum3 : Sum  Inputs=|++
  Processed Accel Data : Outport
  wires:
  Gain1/1 -> Sum3/1
  Data Type Conversion/1 -> Demux/1
  Bias/1 -> Sum3/2, Sum/2, Sum2/2
  Sum2/1 -> Mux/3
  Gain3/1 -> Sum2/1
  Demux/3 -> Gain3/1
  Sum/1 -> Mux/2
  Gain2/1 -> Sum/1
  Demux/2 -> Gain2/1
  Sum3/1 -> Mux/1
  Demux/1 -> Gain1/1
  Raw Accel Data/1 -> Data Type Conversion/1
  Neutral Bias/1 -> Sum1/2
  Mux/1 -> Sum1/1
  Gain/1 -> Processed Accel Data/1
  Sum1/1 -> Gain/1

== system New_Control_Law_I_3Axis/Navigation/Data Conversion and Measurement Calculation/Calculate Gravity Vector/Calibration_GainOffset ==
  Pre : Inport
  Accel_Calib_Gain : Constant  Value=[Accel_Calib_Gain.Gain_X Accel_Calib_Gain.Gain_Y Accel_Calib_Gain.Gain_Z]
      settings: AttributesFormatString=%<Value>
  Accel_Calib_Offset : Constant  Value="[Accel_Calib_Offset.Gain_X  Accel_Calib_Offset.Gain_Y  Accel_Calib_Offset.Gain_Z]"
      settings: AttributesFormatString=%<Value>
  Gain : Gain  Gain=-1  OutDataTypeStr=Inherit: Same as input
  Multiply : Product  Inputs=*/
  Sum : Sum  Inputs=|+-
  Post : Outport
  wires:
  Gain/1 -> Multiply/2
  Accel_Calib_Gain/1 -> Gain/1
  Pre/1 -> Sum/1
  Sum/1 -> Multiply/1
  Accel_Calib_Offset/1 -> Sum/2
  Multiply/1 -> Post/1

== system New_Control_Law_I_3Axis/Navigation/Data Conversion and Measurement Calculation/Calculate Gravity Vector/InitialCondition_Offset ==
  note: For Home Drone
  Pre : Inport
  Accel_Offset : Inport  Port=2
  After : Display
  Before : Display
  Constant2 : Constant  Value=0
  Demux : Demux  Outputs=3
  Demux1 : Demux  Outputs=2
  Gain : Gain
  Gain1 : Gain
  Mux1 : Mux  Inputs=3
  Selector : Selector  InputPortWidth=3  IndexOptions=Index vector (dialog)  Indices=[1 2]  OutputSizes=1
  Sum : Sum  Inputs=|+-
  Sum1 : Sum  Inputs=|+-
  Sum2 : Sum  Inputs=|+-
  Post : Outport
  tag scope: AccelOffset=global
  wires:
  Constant2/1 -> Sum2/2
  Gain1/1 -> Sum1/2
  Gain/1 -> Sum/2
  Selector/1 -> [AccelOffset]
  Pre/1 -> Before/1, Selector/1, Demux/1
  Demux1/2 -> Gain1/1
  Demux1/1 -> Gain/1
  Accel_Offset/1 -> Demux1/1
  Mux1/1 -> After/1, Post/1
  Demux/2 -> Sum1/1
  Demux/1 -> Sum/1
  Sum1/1 -> Mux1/2
  Demux/3 -> Sum2/1
  Sum2/1 -> Mux1/3
  Sum/1 -> Mux1/1

== system New_Control_Law_I_3Axis/Navigation/Data Conversion and Measurement Calculation/Calculate Gravity Vector/Low Pass Filter ==
  Offset Accel : Inport
  Add : Sum
  Gain : Gain  Gain=0.8
  Gain1 : Gain  Gain=0.2
  Unit Delay : UnitDelay  SampleTime=-1
  Filtered Accel : Outport
  wires:
  Offset Accel/1 -> Gain1/1
  Add/1 -> Filtered Accel/1, Unit Delay/1
  Gain/1 -> Add/2
  Gain1/1 -> Add/1
  Unit Delay/1 -> Gain/1

== system New_Control_Law_I_3Axis/Navigation/Data Conversion and Measurement Calculation/Calibration_Scale_and_Offset/Process Raw Mag Data ==
  Magnetometer : Inport
  Process Raw Mag Data (Home_330453) : Subsystem  VariantControl=TempVariantA
  Process Raw Mag Data (Work_255725) : Subsystem  VariantControl=TempVariantB
  MagVector : Outport

== system New_Control_Law_I_3Axis/Navigation/Data Conversion and Measurement Calculation/Remove Offset/Process Raw Rate Gyro Data ==
  note: const float Sensitivity[ 3 ] = { 0.0609 , 0.0609 , 0.0609 } ;
      | const float Neutral[ 3 ] = { 0.0 , 0.0 , 0.0 } ;
      | const int16_t Offset[ 3 ] = { - 73 , 14 , - 13 } ;
      | const int16_t Noises[ 3 ] = { 35 , 35 , 15 } ;
      |
      | int16_t vRaws[ 3 ] = {
      | Navdata :: IMU :: Gyroscope :: getRawX (),
      | Navdata :: IMU :: Gyroscope :: getRawY (),
      | Navdata :: IMU :: Gyroscope :: getRawZ ()
      | } ;
      |
      | gyroscope[i] = vRaws[i] * Gyroscope :: Sensitivity[i] * M_PI / 180.0 ;
  Raw Rate Gyro Data : Inport
  Gain : Gain  Gain=[0.0609, 0.0609, 0.0609]  ParamDataTypeStr=double
  Processed Data : Outport
  wires:
  Gain/1 -> Processed Data/1
  Raw Rate Gyro Data/1 -> Gain/1

== system New_Control_Law_I_3Axis/Navigation/SL3D Visualization/Interchange Axes Mag for SL3D /Home Drone ==
  note: z
  note: x
  note: y
  note: This comes close, however, it doesnt seem that the axis changes properly
      | ie: i rotate drone, the green dot follows it. This  tells me the Z-axis is not
      |  properly placed
  In1 : Inport
  Demux1 : Demux  Outputs=3
  Gain : Gain  Gain=-1
  Gain1 : Gain
  Gain2 : Gain
  Mux2 : Mux  Inputs=3
  Out1 : Outport
  wires:
  Gain1/1 -> Mux2/1
  Demux1/2 -> Gain1/1
  Gain/1 -> Mux2/3
  Demux1/1 -> Gain/1
  Gain2/1 -> Mux2/2
  Demux1/3 -> Gain2/1
  In1/1 -> Demux1/1
  Mux2/1 -> Out1/1

== system New_Control_Law_I_3Axis/Navigation/SL3D Visualization/Interchange Axes Mag for SL3D /Subsystem ==
  note: z
  note: x
  note: y
  note: This comes close, however, it doesnt seem that the axis changes properly
      | ie: i rotate drone, the green dot follows it. This  tells me the Z-axis is not
      |  properly placed
  In1 : Inport
  Demux1 : Demux  Outputs=3
  Gain : Gain
  Gain1 : Gain  Gain=-1
  Gain2 : Gain  Gain=-1
  Mux2 : Mux  Inputs=3
  Out1 : Outport
  wires:
  In1/1 -> Demux1/1
  Demux1/3 -> Gain/1
  Demux1/2 -> Gain1/1
  Mux2/1 -> Out1/1
  Gain1/1 -> Mux2/1
  Gain/1 -> Mux2/3
  Gain2/1 -> Mux2/2
  Demux1/1 -> Gain2/1

== system New_Control_Law_I_3Axis/Navigation/SL3D Visualization/Interchange Axes Mag for SL3D /Work Drone ==
  note: z
  note: x
  note: y
  note: This comes close, however, it doesnt seem that the axis changes properly
      | ie: i rotate drone, the green dot follows it. This  tells me the Z-axis is not
      |  properly placed
  In1 : Inport
  Demux1 : Demux  Outputs=3
  Gain : Gain  Gain=-1
  Gain1 : Gain
  Gain2 : Gain
  Mux2 : Mux  Inputs=3
  Out1 : Outport
  wires:
  Gain1/1 -> Mux2/1
  Demux1/2 -> Gain1/1
  Gain/1 -> Mux2/3
  Demux1/1 -> Gain/1
  Gain2/1 -> Mux2/2
  Demux1/3 -> Gain2/1
  In1/1 -> Demux1/1
  Mux2/1 -> Out1/1

== system New_Control_Law_I_3Axis/Navigation/SL3D Visualization/Interchange Axes Mag for SL3D /Work Drone - supposed work drone .. not really ==
  note: z
  note: x
  note: y
  note: This comes close, however, it doesnt seem that the axis changes properly
      | ie: i rotate drone, the green dot follows it. This  tells me the Z-axis is not
      |  properly placed
  In1 : Inport
  Demux1 : Demux  Outputs=3
  Gain : Gain  Gain=-1
  Gain1 : Gain
  Gain2 : Gain  Gain=-1
  Mux2 : Mux  Inputs=3
  Out1 : Outport
  wires:
  Gain1/1 -> Mux2/1
  Demux1/2 -> Gain1/1
  Gain/1 -> Mux2/3
  Demux1/1 -> Gain/1
  Gain2/1 -> Mux2/2
  Demux1/3 -> Gain2/1
  In1/1 -> Demux1/1
  Mux2/1 -> Out1/1

== system New_Control_Law_I_3Axis/Sensor  Telemetry/CheckSum_Correct_Pressure/CheckSum Correction/Generate Sample Holding Pulse ==
  CheckSumFlag : Inport
  HoldDataTicks_Value : Inport  Port=2
  Chart : Stateflow chart  TreatAsAtomicUnit=on
  Constant2 : Constant
  Logical Operator1 : Logic  AllPortsSameDT=off  OutDataTypeStr=boolean
  Transition Logic Detection : Subsystem
  Hold_Data_Pulse : Outport
  wires:
  Constant2/1 -> Logical Operator1/1
  Logical Operator1/1 -> Hold_Data_Pulse/1
  Chart/1(output) -> Logical Operator1/2
  Transition Logic Detection/1(Transition Detect) -> Chart/1(if_transition)
  CheckSumFlag/1 -> Transition Logic Detection/1(Input)
  HoldDataTicks_Value/1 -> Chart/2(HoldDataTicks)

== system New_Control_Law_I_3Axis/Sensor  Telemetry/CheckSum_Correct_Temp/CheckSum Correction/Generate Sample Holding Pulse ==
  CheckSumFlag : Inport
  HoldDataTicks_Value : Inport  Port=2
  Chart : Stateflow chart  TreatAsAtomicUnit=on
  Constant2 : Constant
  Logical Operator1 : Logic  AllPortsSameDT=off  OutDataTypeStr=boolean
  Transition Logic Detection : Subsystem
  Hold_Data_Pulse : Outport
  wires:
  Constant2/1 -> Logical Operator1/1
  Logical Operator1/1 -> Hold_Data_Pulse/1
  Chart/1(output) -> Logical Operator1/2
  Transition Logic Detection/1(Transition Detect) -> Chart/1(if_transition)
  CheckSumFlag/1 -> Transition Logic Detection/1(Input)
  HoldDataTicks_Value/1 -> Chart/2(HoldDataTicks)

== system New_Control_Law_I_3Axis/Navigation/CheckSum Pre-Processing/Accelerometer Processing/CheckSum Correction/Generate Sample Holding Pulse ==
  CheckSumFlag : Inport
  HoldDataTicks_Value : Inport  Port=2
  Chart : Stateflow chart  TreatAsAtomicUnit=on
  Constant2 : Constant
  Logical Operator1 : Logic  AllPortsSameDT=off  OutDataTypeStr=boolean
  Transition Logic Detection : Subsystem
  Hold_Data_Pulse : Outport
  wires:
  HoldDataTicks_Value/1 -> Chart/2(HoldDataTicks)
  CheckSumFlag/1 -> Transition Logic Detection/1(Input)
  Transition Logic Detection/1(Transition Detect) -> Chart/1(if_transition)
  Chart/1(output) -> Logical Operator1/2
  Logical Operator1/1 -> Hold_Data_Pulse/1
  Constant2/1 -> Logical Operator1/1

== system New_Control_Law_I_3Axis/Navigation/CheckSum Pre-Processing/Magnetometer/CheckSum Correction/Generate Sample Holding Pulse ==
  CheckSumFlag : Inport
  HoldDataTicks_Value : Inport  Port=2
  Chart : Stateflow chart  TreatAsAtomicUnit=on
  Constant2 : Constant
  Logical Operator1 : Logic  AllPortsSameDT=off  OutDataTypeStr=boolean
  Transition Logic Detection : Subsystem
  Hold_Data_Pulse : Outport
  wires:
  HoldDataTicks_Value/1 -> Chart/2(HoldDataTicks)
  CheckSumFlag/1 -> Transition Logic Detection/1(Input)
  Transition Logic Detection/1(Transition Detect) -> Chart/1(if_transition)
  Chart/1(output) -> Logical Operator1/2
  Logical Operator1/1 -> Hold_Data_Pulse/1
  Constant2/1 -> Logical Operator1/1

== system New_Control_Law_I_3Axis/Navigation/CheckSum Pre-Processing/RateGyro Processing/CheckSum Correction/Generate Sample Holding Pulse ==
  CheckSumFlag : Inport
  HoldDataTicks_Value : Inport  Port=2
  Chart : Stateflow chart  TreatAsAtomicUnit=on
  Constant2 : Constant
  Logical Operator1 : Logic  AllPortsSameDT=off  OutDataTypeStr=boolean
  Transition Logic Detection : Subsystem
  Hold_Data_Pulse : Outport
  wires:
  HoldDataTicks_Value/1 -> Chart/2(HoldDataTicks)
  CheckSumFlag/1 -> Transition Logic Detection/1(Input)
  Transition Logic Detection/1(Transition Detect) -> Chart/1(if_transition)
  Chart/1(output) -> Logical Operator1/2
  Logical Operator1/1 -> Hold_Data_Pulse/1
  Constant2/1 -> Logical Operator1/1

== system New_Control_Law_I_3Axis/Navigation/CheckSum Pre-Processing/TempFilter/CheckSum Correction/Generate Sample Holding Pulse ==
  CheckSumFlag : Inport
  HoldDataTicks_Value : Inport  Port=2
  Chart : Stateflow chart  TreatAsAtomicUnit=on
  Constant2 : Constant
  Logical Operator1 : Logic  AllPortsSameDT=off  OutDataTypeStr=boolean
  Transition Logic Detection : Subsystem
  Hold_Data_Pulse : Outport
  wires:
  HoldDataTicks_Value/1 -> Chart/2(HoldDataTicks)
  CheckSumFlag/1 -> Transition Logic Detection/1(Input)
  Transition Logic Detection/1(Transition Detect) -> Chart/1(if_transition)
  Chart/1(output) -> Logical Operator1/2
  Logical Operator1/1 -> Hold_Data_Pulse/1
  Constant2/1 -> Logical Operator1/1

== system New_Control_Law_I_3Axis/Navigation/CheckSum Pre-Processing/Ultrasound Processing/CheckSum Correction/Generate Sample Holding Pulse ==
  CheckSumFlag : Inport
  HoldDataTicks_Value : Inport  Port=2
  Chart : Stateflow chart  TreatAsAtomicUnit=on
  Constant2 : Constant
  Logical Operator1 : Logic  AllPortsSameDT=off  OutDataTypeStr=boolean
  Transition Logic Detection : Subsystem
  Hold_Data_Pulse : Outport
  wires:
  HoldDataTicks_Value/1 -> Chart/2(HoldDataTicks)
  CheckSumFlag/1 -> Transition Logic Detection/1(Input)
  Transition Logic Detection/1(Transition Detect) -> Chart/1(if_transition)
  Chart/1(output) -> Logical Operator1/2
  Logical Operator1/1 -> Hold_Data_Pulse/1
  Constant2/1 -> Logical Operator1/1

== system New_Control_Law_I_3Axis/Navigation/Data Conversion and Measurement Calculation/Calibration_Scale_and_Offset/Process Raw Mag Data/Process Raw Mag Data (Home_330453) ==
  note: magnetometer[ 0 ] = - ( float ) navdata.mx ;
      | magnetometer[ 1 ] = ( float ) navdata.my ;
      | magnetometer[ 2 ] = - ( float ) navdata.mz ;
      | const float Sensitivity[ 3 ] = { 0.0071492608 , 0.0070882491 , 0.0074057781 } ;
      | const float Neutral[ 3 ] = { 118.0 , - 65.0 , 110.0 } ;
  Magnetometer : Inport
  Bias : Constant  Commented=on  Value=[-23 4.3 1.44]
  Constant : Constant  Value=[Mag_Calib_Offset_Vector.Gain_X Mag_Calib_Offset_Vector.Gain_Y Mag_Calib_Offset_Vector.Gain_Z]
      settings: AttributesFormatString=%<Value>
  Constant1 : Constant  Value=[Mag_Calib_Gain_Vector.Gain_X Mag_Calib_Gain_Vector.Gain_Y Mag_Calib_Gain_Vector.Gain_Z]
      settings: AttributesFormatString=%<Value>
  Divide : Product  Inputs=/*
  Sum : Sum  Inputs=|+-
  postGain : Gain  Commented=on  Gain=1./[187 163 139]
  MagVector : Outport
  wires:
  Constant1/1 -> Divide/1
  Sum/1 -> Divide/2
  Magnetometer/1 -> Sum/1
  Constant/1 -> Sum/2
  Divide/1 -> MagVector/1

== system New_Control_Law_I_3Axis/Navigation/Data Conversion and Measurement Calculation/Calibration_Scale_and_Offset/Process Raw Mag Data/Process Raw Mag Data (Work_255725) ==
  note: 158 145 136
  note: magnetometer[ 0 ] = - ( float ) navdata.mx ;
      | magnetometer[ 1 ] = ( float ) navdata.my ;
      | magnetometer[ 2 ] = - ( float ) navdata.mz ;
      | const float Sensitivity[ 3 ] = { 0.0071492608 , 0.0070882491 , 0.0074057781 } ;
      | const float Neutral[ 3 ] = { 118.0 , - 65.0 , 110.0 } ;
  Magnetometer : Inport
  Bias : Constant  Value=[2.93 18.9 77.5]
  Low Pass Filter1 : Subsystem  Commented=through
      mask Display: disp(['Elliptic Filter with 20 Hz corner', '\n', '44 dB stopband.'])
  Sum : Sum  Inputs=|+-
  postGain : Gain  Gain=1./[167 135 132]
  preGain : Gain  Commented=through  Gain=[1 1 1]
  MagVector : Outport
  wires:
  postGain/1 -> Low Pass Filter1/1(Input)
  Magnetometer/1 -> preGain/1
  Sum/1 -> postGain/1
  preGain/1 -> Sum/1
  Bias/1 -> Sum/2
  Low Pass Filter1/1(Output) -> MagVector/1
